simulink model "general_charger_2_precharge"  (R2013a)
settings: Solver=ode23  StartTime=0  StopTime=1.5  RelTol=1e-3
PreLoadFcn:
  | Ts =5e-6;
values from neighbouring files (symbols this model uses):
  ac_volt = 169    [charger_init.m]    (also in charger_init_simpl.m)
  acdc_on_time = 0.2    [charger_init.m]    (also in charger_init_simpl.m = 0)
  Cdc = 2e-3    (= 0.002)    [charger_init.m]    (also in charger_init_simpl.m)
  dcAd = dcinvexp*(eye(dcnstates) + (Ts/2)*dcAc)    [charger_init.m]    (also in charger_init_simpl.m)
  dcBd = dcinvexp*dcBc    [charger_init.m]    (also in charger_init_simpl.m)
  dcCd = dcCc*dcinvexp*Ts    [charger_init.m]    (also in charger_init_simpl.m)
  dcDd = dcCc*dcinvexp*dcBc*(Ts/2) + dcDc    [charger_init.m]    (also in charger_init_simpl.m)
  ESRCd = 70e-3    (= 0.07)    [charger_init.m]    (also in charger_init_simpl.m)
  ESRLdcdc = 0.1    [charger_init.m]    (also in charger_init_simpl.m)
  ESRLin = 0.2    [charger_init.m]    (also in charger_init_simpl.m = 0.1)
  Ldcdc = 1.3e-3    (= 0.0013)    [charger_init.m]    (also in charger_init_simpl.m = 0.0014)
  Lin = 1.5e-3    (= 0.0015)    [charger_init.m]    (also in charger_init_simpl.m = 0.001)
  P = 1.92e3    (= 1920)    [charger_init.m]    (also in charger_init_simpl.m)
  pre_charge_off = 0.2    [charger_init.m]
  pre_charge_r = 10    [charger_init.m]    (also in charger_init_simpl.m = 6)
  pre_charge_ramp = (dc_volt - Vdcmin)/(acdc_ramp_end_time - acdc_on_time)    (= 336.666666667)    [charger_init.m]    (also in charger_init_simpl.m = (dc_volt - Vdcmin)/(acdc_ramp_end_time - acdc_on_time))
  Q = 0    [charger_init.m]    (also in charger_init_simpl.m)
  Rbatt = 0.20    (= 0.2)    [charger_init.m]    (also in charger_init_simpl.m = 0.1)
  switch_Ts = 5e-5    (= 5e-05)    [charger_init.m]    (also in charger_init_simpl.m)
  sys_Ts = 5e-6    (= 5e-06)    [charger_init.m]    (also in charger_init_simpl.m)
  Vdcmin = ac_volt + 10    (= 179)    [charger_init.m]    (also in charger_init_simpl.m)
  voc = 105    [charger_init.m]    (also in charger_init_simpl.m)
undefined symbols (not defined in the file or in its folder): cpi
undefined symbols (not defined in the file): active_power_on, Ad, Bd, Cd, dc_volt, dcdc_cc_ref, dcdc_cv_ref, dcdc_iki, dcdc_ikp, dcdc_on, dcdc_vki, dcdc_vkp, Dd, dq_id_ki, dq_id_kp, dq_iq_ki, dq_iq_kp, dq_vdc_ki, dq_vdc_kp, dqQ_ki, dqQ_kp, P_ki, P_kp, pi_iac_ki, pi_iac_kp, pi_vdc_ki, pi_vdc_kp, piQ_ki, piQ_kp, pr_iac_kp, pr_pr_ki, pr_pr_kp, pr_vdc_ki, pr_vdc_kp, reactive_power_on
libraries: simulink_extras x165, powerlib x64, simulink x35, powerlib_meascontrol x11
(part 4 of 7)

== system general_charger_2_precharge/Measurements/THD/discrete low pass filter1/Ad(2,2) ==
  in : Inport
  Constant1 : Constant  Value=variable
  Product1 : Product
  Scope1 : Scope  NumInputPorts=2
      settings: YMin=-5~-5  YMax=5~5
  q rounder16 : Subsystem  mask{q=nQ, range=maxRange}
      mask prompts: q "q value"; range "q range"
  out : Outport
  wires:
  q rounder16/1(out) -> Product1/1, Scope1/2
  Constant1/1 -> Scope1/1, q rounder16/1(in)
  Product1/1 -> out/1
  in/1 -> Product1/2

== system general_charger_2_precharge/Measurements/THD/discrete low pass filter1/Ad(2,3) ==
  in : Inport
  Constant1 : Constant  Value=variable
  Product1 : Product
  Scope1 : Scope  NumInputPorts=2
      settings: YMin=-5~-5  YMax=5~5
  q rounder16 : Subsystem  mask{q=nQ, range=maxRange}
      mask prompts: q "q value"; range "q range"
  out : Outport
  wires:
  q rounder16/1(out) -> Product1/1, Scope1/2
  Constant1/1 -> Scope1/1, q rounder16/1(in)
  Product1/1 -> out/1
  in/1 -> Product1/2

== system general_charger_2_precharge/Measurements/THD/discrete low pass filter1/Ad(3,1) ==
  in : Inport
  Constant1 : Constant  Value=variable
  Product1 : Product
  Scope1 : Scope  NumInputPorts=2
      settings: YMin=-5~-5  YMax=5~5
  q rounder16 : Subsystem  mask{q=nQ, range=maxRange}
      mask prompts: q "q value"; range "q range"
  out : Outport
  wires:
  q rounder16/1(out) -> Product1/1, Scope1/2
  Constant1/1 -> Scope1/1, q rounder16/1(in)
  Product1/1 -> out/1
  in/1 -> Product1/2

== system general_charger_2_precharge/Measurements/THD/discrete low pass filter1/Ad(3,2) ==
  in : Inport
  Constant1 : Constant  Value=variable
  Product1 : Product
  Scope1 : Scope  NumInputPorts=2
      settings: YMin=-5~-5  YMax=5~5
  q rounder16 : Subsystem  mask{q=nQ, range=maxRange}
      mask prompts: q "q value"; range "q range"
  out : Outport
  wires:
  q rounder16/1(out) -> Product1/1, Scope1/2
  Constant1/1 -> Scope1/1, q rounder16/1(in)
  Product1/1 -> out/1
  in/1 -> Product1/2

== system general_charger_2_precharge/Measurements/THD/discrete low pass filter1/Ad(3,3) ==
  in : Inport
  Constant1 : Constant  Value=variable
  Product1 : Product
  Scope1 : Scope  NumInputPorts=2
      settings: YMin=-5~-5  YMax=5~5
  q rounder16 : Subsystem  mask{q=nQ, range=maxRange}
      mask prompts: q "q value"; range "q range"
  out : Outport
  wires:
  q rounder16/1(out) -> Product1/1, Scope1/2
  Constant1/1 -> Scope1/1, q rounder16/1(in)
  Product1/1 -> out/1
  in/1 -> Product1/2

== system general_charger_2_precharge/Measurements/THD/discrete low pass filter1/Bd(1) ==
  in : Inport
  Constant1 : Constant  Value=variable
  Product1 : Product
  q rounder16 : Subsystem  mask{q=nQ, range=maxRange}
      mask prompts: q "q value"; range "q range"
  out : Outport
  wires:
  q rounder16/1(out) -> Product1/1
  Constant1/1 -> q rounder16/1(in)
  Product1/1 -> out/1
  in/1 -> Product1/2

== system general_charger_2_precharge/Measurements/THD/discrete low pass filter1/Bd(2) ==
  in : Inport
  Constant1 : Constant  Value=variable
  Product1 : Product
  q rounder16 : Subsystem  mask{q=nQ, range=maxRange}
      mask prompts: q "q value"; range "q range"
  out : Outport
  wires:
  q rounder16/1(out) -> Product1/1
  Constant1/1 -> q rounder16/1(in)
  Product1/1 -> out/1
  in/1 -> Product1/2

== system general_charger_2_precharge/Measurements/THD/discrete low pass filter1/Bd(3) ==
  in : Inport
  Constant1 : Constant  Value=variable
  Product1 : Product
  q rounder16 : Subsystem  mask{q=nQ, range=maxRange}
      mask prompts: q "q value"; range "q range"
  out : Outport
  wires:
  q rounder16/1(out) -> Product1/1
  Constant1/1 -> q rounder16/1(in)
  Product1/1 -> out/1
  in/1 -> Product1/2

== system general_charger_2_precharge/Measurements/THD/discrete low pass filter1/Cd(1) ==
  in : Inport
  Constant1 : Constant  Value=variable
  Product1 : Product
  q rounder16 : Subsystem  mask{q=nQ, range=maxRange}
      mask prompts: q "q value"; range "q range"
  out : Outport
  wires:
  q rounder16/1(out) -> Product1/1
  Constant1/1 -> q rounder16/1(in)
  Product1/1 -> out/1
  in/1 -> Product1/2

== system general_charger_2_precharge/Measurements/THD/discrete low pass filter1/Cd(2) ==
  in : Inport
  Constant1 : Constant  Value=variable
  Product1 : Product
  q rounder16 : Subsystem  mask{q=nQ, range=maxRange}
      mask prompts: q "q value"; range "q range"
  out : Outport
  wires:
  q rounder16/1(out) -> Product1/1
  Constant1/1 -> q rounder16/1(in)
  Product1/1 -> out/1
  in/1 -> Product1/2

== system general_charger_2_precharge/Measurements/THD/discrete low pass filter1/Cd(3) ==
  in : Inport
  Constant1 : Constant  Value=variable
  Product1 : Product
  q rounder16 : Subsystem  mask{q=nQ, range=maxRange}
      mask prompts: q "q value"; range "q range"
  out : Outport
  wires:
  q rounder16/1(out) -> Product1/1
  Constant1/1 -> q rounder16/1(in)
  Product1/1 -> out/1
  in/1 -> Product1/2

== system general_charger_2_precharge/Measurements/THD/discrete low pass filter1/Dd ==
  in : Inport
  Constant1 : Constant  Value=variable
  Product1 : Product
  Scope1 : Scope  NumInputPorts=2
      settings: YMin=-5~-5  YMax=5~5
  q rounder16 : Subsystem  mask{q=nQ, range=maxRange}
      mask prompts: q "q value"; range "q range"
  out : Outport
  wires:
  q rounder16/1(out) -> Product1/1, Scope1/2
  Constant1/1 -> Scope1/1, q rounder16/1(in)
  Product1/1 -> out/1
  in/1 -> Product1/2

== system general_charger_2_precharge/Measurements/THD/discrete low pass filter1/q rounder1 ==
  in : Inport
  Gain9 : Gain  Gain=2^-q
  Idealized ADC quantizer : simulink_extras/Additional Discrete/Idealized ADC quantizer  NumberOfConverterBits=32  Vmin=-range  Vmax=range  OutputDataType=double  OutputNegativeValues=on
  out : Outport
  wires:
  in/1 -> Idealized ADC quantizer/1
  Idealized ADC quantizer/1 -> Gain9/1
  Gain9/1 -> out/1

== system general_charger_2_precharge/Measurements/THD/discrete low pass filter1/q rounder10 ==
  in : Inport
  Gain9 : Gain  Gain=2^-q
  Idealized ADC quantizer : simulink_extras/Additional Discrete/Idealized ADC quantizer  NumberOfConverterBits=32  Vmin=-range  Vmax=range  OutputDataType=double  OutputNegativeValues=on
  out : Outport
  wires:
  in/1 -> Idealized ADC quantizer/1
  Idealized ADC quantizer/1 -> Gain9/1
  Gain9/1 -> out/1

== system general_charger_2_precharge/Measurements/THD/discrete low pass filter1/q rounder11 ==
  in : Inport
  Gain9 : Gain  Gain=2^-q
  Idealized ADC quantizer : simulink_extras/Additional Discrete/Idealized ADC quantizer  NumberOfConverterBits=32  Vmin=-range  Vmax=range  OutputDataType=double  OutputNegativeValues=on
  out : Outport
  wires:
  in/1 -> Idealized ADC quantizer/1
  Idealized ADC quantizer/1 -> Gain9/1
  Gain9/1 -> out/1

== system general_charger_2_precharge/Measurements/THD/discrete low pass filter1/q rounder12 ==
  in : Inport
  Gain9 : Gain  Gain=2^-q
  Idealized ADC quantizer : simulink_extras/Additional Discrete/Idealized ADC quantizer  NumberOfConverterBits=32  Vmin=-range  Vmax=range  OutputDataType=double  OutputNegativeValues=on
  out : Outport
  wires:
  in/1 -> Idealized ADC quantizer/1
  Idealized ADC quantizer/1 -> Gain9/1
  Gain9/1 -> out/1

== system general_charger_2_precharge/Measurements/THD/discrete low pass filter1/q rounder13 ==
  in : Inport
  Gain9 : Gain  Gain=2^-q
  Idealized ADC quantizer : simulink_extras/Additional Discrete/Idealized ADC quantizer  NumberOfConverterBits=32  Vmin=-range  Vmax=range  OutputDataType=double  OutputNegativeValues=on
  out : Outport
  wires:
  in/1 -> Idealized ADC quantizer/1
  Idealized ADC quantizer/1 -> Gain9/1
  Gain9/1 -> out/1

== system general_charger_2_precharge/Measurements/THD/discrete low pass filter1/q rounder14 ==
  in : Inport
  Gain9 : Gain  Gain=2^-q
  Idealized ADC quantizer : simulink_extras/Additional Discrete/Idealized ADC quantizer  NumberOfConverterBits=32  Vmin=-range  Vmax=range  OutputDataType=double  OutputNegativeValues=on
  out : Outport
  wires:
  in/1 -> Idealized ADC quantizer/1
  Idealized ADC quantizer/1 -> Gain9/1
  Gain9/1 -> out/1

== system general_charger_2_precharge/Measurements/THD/discrete low pass filter1/q rounder15 ==
  in : Inport
  Gain9 : Gain  Gain=2^-q
  Idealized ADC quantizer : simulink_extras/Additional Discrete/Idealized ADC quantizer  NumberOfConverterBits=32  Vmin=-range  Vmax=range  OutputDataType=double  OutputNegativeValues=on
  out : Outport
  wires:
  in/1 -> Idealized ADC quantizer/1
  Idealized ADC quantizer/1 -> Gain9/1
  Gain9/1 -> out/1

== system general_charger_2_precharge/Measurements/THD/discrete low pass filter1/q rounder16 ==
  in : Inport
  Gain9 : Gain  Gain=2^-q
  Idealized ADC quantizer : simulink_extras/Additional Discrete/Idealized ADC quantizer  NumberOfConverterBits=32  Vmin=-range  Vmax=range  OutputDataType=double  OutputNegativeValues=on
  out : Outport
  wires:
  in/1 -> Idealized ADC quantizer/1
  Idealized ADC quantizer/1 -> Gain9/1
  Gain9/1 -> out/1

== system general_charger_2_precharge/Measurements/THD/discrete low pass filter1/q rounder17 ==
  in : Inport
  Gain9 : Gain  Gain=2^-q
  Idealized ADC quantizer : simulink_extras/Additional Discrete/Idealized ADC quantizer  NumberOfConverterBits=32  Vmin=-range  Vmax=range  OutputDataType=double  OutputNegativeValues=on
  out : Outport
  wires:
  in/1 -> Idealized ADC quantizer/1
  Idealized ADC quantizer/1 -> Gain9/1
  Gain9/1 -> out/1

== system general_charger_2_precharge/Measurements/THD/discrete low pass filter1/q rounder2 ==
  in : Inport
  Gain9 : Gain  Gain=2^-q
  Idealized ADC quantizer : simulink_extras/Additional Discrete/Idealized ADC quantizer  NumberOfConverterBits=32  Vmin=-range  Vmax=range  OutputDataType=double  OutputNegativeValues=on
  out : Outport
  wires:
  in/1 -> Idealized ADC quantizer/1
  Idealized ADC quantizer/1 -> Gain9/1
  Gain9/1 -> out/1

== system general_charger_2_precharge/Measurements/THD/discrete low pass filter1/q rounder3 ==
  in : Inport
  Gain9 : Gain  Gain=2^-q
  Idealized ADC quantizer : simulink_extras/Additional Discrete/Idealized ADC quantizer  NumberOfConverterBits=32  Vmin=-range  Vmax=range  OutputDataType=double  OutputNegativeValues=on
  out : Outport
  wires:
  in/1 -> Idealized ADC quantizer/1
  Idealized ADC quantizer/1 -> Gain9/1
  Gain9/1 -> out/1

== system general_charger_2_precharge/Measurements/THD/discrete low pass filter1/q rounder4 ==
  in : Inport
  Gain9 : Gain  Gain=2^-q
  Idealized ADC quantizer : simulink_extras/Additional Discrete/Idealized ADC quantizer  NumberOfConverterBits=32  Vmin=-range  Vmax=range  OutputDataType=double  OutputNegativeValues=on
  out : Outport
  wires:
  in/1 -> Idealized ADC quantizer/1
  Idealized ADC quantizer/1 -> Gain9/1
  Gain9/1 -> out/1

== system general_charger_2_precharge/Measurements/THD/discrete low pass filter1/q rounder5 ==
  in : Inport
  Gain9 : Gain  Gain=2^-q
  Idealized ADC quantizer : simulink_extras/Additional Discrete/Idealized ADC quantizer  NumberOfConverterBits=32  Vmin=-range  Vmax=range  OutputDataType=double  OutputNegativeValues=on
  out : Outport
  wires:
  in/1 -> Idealized ADC quantizer/1
  Idealized ADC quantizer/1 -> Gain9/1
  Gain9/1 -> out/1

== system general_charger_2_precharge/Measurements/THD/discrete low pass filter1/q rounder6 ==
  in : Inport
  Gain9 : Gain  Gain=2^-q
  Idealized ADC quantizer : simulink_extras/Additional Discrete/Idealized ADC quantizer  NumberOfConverterBits=32  Vmin=-range  Vmax=range  OutputDataType=double  OutputNegativeValues=on
  out : Outport
  wires:
  in/1 -> Idealized ADC quantizer/1
  Idealized ADC quantizer/1 -> Gain9/1
  Gain9/1 -> out/1

== system general_charger_2_precharge/Measurements/THD/discrete low pass filter1/q rounder7 ==
  in : Inport
  Gain9 : Gain  Gain=2^-q
  Idealized ADC quantizer : simulink_extras/Additional Discrete/Idealized ADC quantizer  NumberOfConverterBits=32  Vmin=-range  Vmax=range  OutputDataType=double  OutputNegativeValues=on
  out : Outport
  wires:
  in/1 -> Idealized ADC quantizer/1
  Idealized ADC quantizer/1 -> Gain9/1
  Gain9/1 -> out/1

== system general_charger_2_precharge/Measurements/THD/discrete low pass filter1/q rounder8 ==
  in : Inport
  Gain9 : Gain  Gain=2^-q
  Idealized ADC quantizer : simulink_extras/Additional Discrete/Idealized ADC quantizer  NumberOfConverterBits=32  Vmin=-range  Vmax=range  OutputDataType=double  OutputNegativeValues=on
  out : Outport
  wires:
  in/1 -> Idealized ADC quantizer/1
  Idealized ADC quantizer/1 -> Gain9/1
  Gain9/1 -> out/1

== system general_charger_2_precharge/Measurements/THD/discrete low pass filter1/q rounder9 ==
  in : Inport
  Gain9 : Gain  Gain=2^-q
  Idealized ADC quantizer : simulink_extras/Additional Discrete/Idealized ADC quantizer  NumberOfConverterBits=32  Vmin=-range  Vmax=range  OutputDataType=double  OutputNegativeValues=on
  out : Outport
  wires:
  in/1 -> Idealized ADC quantizer/1
  Idealized ADC quantizer/1 -> Gain9/1
  Gain9/1 -> out/1

== system general_charger_2_precharge/Measurements/discrete low pass filter1/Ad(1,1)/q rounder16 ==
  in : Inport
  Gain9 : Gain  Gain=2^-q
  Idealized ADC quantizer : simulink_extras/Additional Discrete/Idealized ADC quantizer  NumberOfConverterBits=32  Vmin=-range  Vmax=range  OutputDataType=double  OutputNegativeValues=on
  out : Outport
  wires:
  in/1 -> Idealized ADC quantizer/1
  Idealized ADC quantizer/1 -> Gain9/1
  Gain9/1 -> out/1

== system general_charger_2_precharge/Measurements/discrete low pass filter1/Ad(1,2)/q rounder16 ==
  in : Inport
  Gain9 : Gain  Gain=2^-q
  Idealized ADC quantizer : simulink_extras/Additional Discrete/Idealized ADC quantizer  NumberOfConverterBits=32  Vmin=-range  Vmax=range  OutputDataType=double  OutputNegativeValues=on
  out : Outport
  wires:
  in/1 -> Idealized ADC quantizer/1
  Idealized ADC quantizer/1 -> Gain9/1
  Gain9/1 -> out/1

== system general_charger_2_precharge/Measurements/discrete low pass filter1/Ad(1,3)/q rounder16 ==
  in : Inport
  Gain9 : Gain  Gain=2^-q
  Idealized ADC quantizer : simulink_extras/Additional Discrete/Idealized ADC quantizer  NumberOfConverterBits=32  Vmin=-range  Vmax=range  OutputDataType=double  OutputNegativeValues=on
  out : Outport
  wires:
  in/1 -> Idealized ADC quantizer/1
  Idealized ADC quantizer/1 -> Gain9/1
  Gain9/1 -> out/1

== system general_charger_2_precharge/Measurements/discrete low pass filter1/Ad(2,1)/q rounder16 ==
  in : Inport
  Gain9 : Gain  Gain=2^-q
  Idealized ADC quantizer : simulink_extras/Additional Discrete/Idealized ADC quantizer  NumberOfConverterBits=32  Vmin=-range  Vmax=range  OutputDataType=double  OutputNegativeValues=on
  out : Outport
  wires:
  in/1 -> Idealized ADC quantizer/1
  Idealized ADC quantizer/1 -> Gain9/1
  Gain9/1 -> out/1

== system general_charger_2_precharge/Measurements/discrete low pass filter1/Ad(2,2)/q rounder16 ==
  in : Inport
  Gain9 : Gain  Gain=2^-q
  Idealized ADC quantizer : simulink_extras/Additional Discrete/Idealized ADC quantizer  NumberOfConverterBits=32  Vmin=-range  Vmax=range  OutputDataType=double  OutputNegativeValues=on
  out : Outport
  wires:
  in/1 -> Idealized ADC quantizer/1
  Idealized ADC quantizer/1 -> Gain9/1
  Gain9/1 -> out/1

== system general_charger_2_precharge/Measurements/discrete low pass filter1/Ad(2,3)/q rounder16 ==
  in : Inport
  Gain9 : Gain  Gain=2^-q
  Idealized ADC quantizer : simulink_extras/Additional Discrete/Idealized ADC quantizer  NumberOfConverterBits=32  Vmin=-range  Vmax=range  OutputDataType=double  OutputNegativeValues=on
  out : Outport
  wires:
  in/1 -> Idealized ADC quantizer/1
  Idealized ADC quantizer/1 -> Gain9/1
  Gain9/1 -> out/1

== system general_charger_2_precharge/Measurements/discrete low pass filter1/Ad(3,1)/q rounder16 ==
  in : Inport
  Gain9 : Gain  Gain=2^-q
  Idealized ADC quantizer : simulink_extras/Additional Discrete/Idealized ADC quantizer  NumberOfConverterBits=32  Vmin=-range  Vmax=range  OutputDataType=double  OutputNegativeValues=on
  out : Outport
  wires:
  in/1 -> Idealized ADC quantizer/1
  Idealized ADC quantizer/1 -> Gain9/1
  Gain9/1 -> out/1

== system general_charger_2_precharge/Measurements/discrete low pass filter1/Ad(3,2)/q rounder16 ==
  in : Inport
  Gain9 : Gain  Gain=2^-q
  Idealized ADC quantizer : simulink_extras/Additional Discrete/Idealized ADC quantizer  NumberOfConverterBits=32  Vmin=-range  Vmax=range  OutputDataType=double  OutputNegativeValues=on
  out : Outport
  wires:
  in/1 -> Idealized ADC quantizer/1
  Idealized ADC quantizer/1 -> Gain9/1
  Gain9/1 -> out/1

== system general_charger_2_precharge/Measurements/discrete low pass filter1/Ad(3,3)/q rounder16 ==
  in : Inport
  Gain9 : Gain  Gain=2^-q
  Idealized ADC quantizer : simulink_extras/Additional Discrete/Idealized ADC quantizer  NumberOfConverterBits=32  Vmin=-range  Vmax=range  OutputDataType=double  OutputNegativeValues=on
  out : Outport
  wires:
  in/1 -> Idealized ADC quantizer/1
  Idealized ADC quantizer/1 -> Gain9/1
  Gain9/1 -> out/1

== system general_charger_2_precharge/Measurements/discrete low pass filter1/Bd(1)/q rounder16 ==
  in : Inport
  Gain9 : Gain  Gain=2^-q
  Idealized ADC quantizer : simulink_extras/Additional Discrete/Idealized ADC quantizer  NumberOfConverterBits=32  Vmin=-range  Vmax=range  OutputDataType=double  OutputNegativeValues=on
  out : Outport
  wires:
  in/1 -> Idealized ADC quantizer/1
  Idealized ADC quantizer/1 -> Gain9/1
  Gain9/1 -> out/1

== system general_charger_2_precharge/Measurements/discrete low pass filter1/Bd(2)/q rounder16 ==
  in : Inport
  Gain9 : Gain  Gain=2^-q
  Idealized ADC quantizer : simulink_extras/Additional Discrete/Idealized ADC quantizer  NumberOfConverterBits=32  Vmin=-range  Vmax=range  OutputDataType=double  OutputNegativeValues=on
  out : Outport
  wires:
  in/1 -> Idealized ADC quantizer/1
  Idealized ADC quantizer/1 -> Gain9/1
  Gain9/1 -> out/1

== system general_charger_2_precharge/Measurements/discrete low pass filter1/Bd(3)/q rounder16 ==
  in : Inport
  Gain9 : Gain  Gain=2^-q
  Idealized ADC quantizer : simulink_extras/Additional Discrete/Idealized ADC quantizer  NumberOfConverterBits=32  Vmin=-range  Vmax=range  OutputDataType=double  OutputNegativeValues=on
  out : Outport
  wires:
  in/1 -> Idealized ADC quantizer/1
  Idealized ADC quantizer/1 -> Gain9/1
  Gain9/1 -> out/1

== system general_charger_2_precharge/Measurements/discrete low pass filter1/Cd(1)/q rounder16 ==
  in : Inport
  Gain9 : Gain  Gain=2^-q
  Idealized ADC quantizer : simulink_extras/Additional Discrete/Idealized ADC quantizer  NumberOfConverterBits=32  Vmin=-range  Vmax=range  OutputDataType=double  OutputNegativeValues=on
  out : Outport
  wires:
  in/1 -> Idealized ADC quantizer/1
  Idealized ADC quantizer/1 -> Gain9/1
  Gain9/1 -> out/1

== system general_charger_2_precharge/Measurements/discrete low pass filter1/Cd(2)/q rounder16 ==
  in : Inport
  Gain9 : Gain  Gain=2^-q
  Idealized ADC quantizer : simulink_extras/Additional Discrete/Idealized ADC quantizer  NumberOfConverterBits=32  Vmin=-range  Vmax=range  OutputDataType=double  OutputNegativeValues=on
  out : Outport
  wires:
  in/1 -> Idealized ADC quantizer/1
  Idealized ADC quantizer/1 -> Gain9/1
  Gain9/1 -> out/1

== system general_charger_2_precharge/Measurements/discrete low pass filter1/Cd(3)/q rounder16 ==
  in : Inport
  Gain9 : Gain  Gain=2^-q
  Idealized ADC quantizer : simulink_extras/Additional Discrete/Idealized ADC quantizer  NumberOfConverterBits=32  Vmin=-range  Vmax=range  OutputDataType=double  OutputNegativeValues=on
  out : Outport
  wires:
  in/1 -> Idealized ADC quantizer/1
  Idealized ADC quantizer/1 -> Gain9/1
  Gain9/1 -> out/1

== system general_charger_2_precharge/Measurements/discrete low pass filter1/Dd/q rounder16 ==
  in : Inport
  Gain9 : Gain  Gain=2^-q
  Idealized ADC quantizer : simulink_extras/Additional Discrete/Idealized ADC quantizer  NumberOfConverterBits=32  Vmin=-range  Vmax=range  OutputDataType=double  OutputNegativeValues=on
  out : Outport
  wires:
  in/1 -> Idealized ADC quantizer/1
  Idealized ADC quantizer/1 -> Gain9/1
  Gain9/1 -> out/1

== system general_charger_2_precharge/control_stage/AC//DC Control/DQ Controller/AB-DQ Transform ==
  Va : Inport
  Ia : Inport  Port=2
  phi : Inport  Port=3
  AB->DQ : Subsystem  mask{abdq_f=60, abdq_Ts=switch_Ts}
      mask prompts: abdq_f "frequency"; abdq_Ts "Sample Time"
      mask init:
      | SpC=1/abdq_f/4/abdq_Ts;
      | RSpC=ceil(SpC);
  PLL : Subsystem  mask{pll_f=60, pll_Ts=switch_Ts, pll_ki=50, pll_kp=5}
      mask prompts: pll_f "frequency"; pll_Ts "Sample Time"; pll_ki "PI Integral Gain"; pll_kp "PI Proportional Gain"
  Vd : Outport
  Vq : Outport  Port=2
  Id : Outport  Port=3
  Iq : Outport  Port=4
  theta : Outport  Port=5
  wires:
  phi/1 -> AB->DQ/3(phi)
  Va/1 -> PLL/1(signal_in)
  Ia/1 -> AB->DQ/1(A)
  PLL/2(D) -> Vd/1
  PLL/3(Q) -> Vq/1
  PLL/1(angle_out) -> theta/1, AB->DQ/2(wt)
  AB->DQ/1(D) -> Id/1
  AB->DQ/2(Q) -> Iq/1

== system general_charger_2_precharge/control_stage/AC//DC Control/DQ Controller/DQ Controller Submodule ==
  note: id_error
  Vdc : Inport
  Vd : Inport  Port=2
  Id : Inport  Port=3
  Iq : Inport  Port=4
  Vwt : Inport  Port=5
  Add{1..2,6..7} (4 alike) : Sum  Inputs=-+
  Add3 : Sum  Inputs=+-
  Add4 : Sum  Inputs=+++
  Add5 : Sum  Inputs=+-
  Constant : Constant  Value=50
  Constant4 : Constant  Value=vdc
  DQ-->A : Subsystem
  Divide : Product  Inputs=*/
  Divide1 : Product  Inputs=/*
  Gain : Gain  Gain=2*pi*f*L
  Gain1 : Gain  Gain=R
  Gain2 : Gain  Gain=2*pi*f*L
  Gain3 : Gain  Gain=R
  PI1 : Subsystem  mask{ki=id_ki, kp=id_kp, Ts_pi=Ts, int_sat_up=500, int_sat_low=-500, pi_sat_up=500, pi_sat_low=-500}
      mask prompts: ki "Integral Gain"; kp "Proportional Gain"; Ts_pi "Sample Time"; int_sat_up "Integral Saturation Upper"; int_sat_low "Integral Saturation Lower"; pi_sat_up "PI Controller Saturation Upper"; pi_sat_low "PI Controller Saturation Lower"
      mask Display: disp('PI')
  PI2 : Subsystem  mask{ki=vdc_ki, kp=vdc_kp, Ts_pi=Ts, int_sat_up=500, int_sat_low=-500, pi_sat_up=500, pi_sat_low=-500}
      mask prompts: ki "Integral Gain"; kp "Proportional Gain"; Ts_pi "Sample Time"; int_sat_up "Integral Saturation Upper"; int_sat_low "Integral Saturation Lower"; pi_sat_up "PI Controller Saturation Upper"; pi_sat_low "PI Controller Saturation Lower"
      mask Display: disp('PI')
  PI3 : Subsystem  mask{ki=iq_ki, kp=iq_kp, Ts_pi=Ts, int_sat_up=500, int_sat_low=-500, pi_sat_up=500, pi_sat_low=-500}
      mask prompts: ki "Integral Gain"; kp "Proportional Gain"; Ts_pi "Sample Time"; int_sat_up "Integral Saturation Upper"; int_sat_low "Integral Saturation Lower"; pi_sat_up "PI Controller Saturation Upper"; pi_sat_low "PI Controller Saturation Lower"
      mask Display: disp('PI')
  Ramp : simulink/Sources/Ramp  slope=pre_charge_ramp  start=acdc_on_time  X0=Vdcmin
  Reactive Power Control Module : Subsystem
  Scope : Scope
      settings: SaveName=ScopeData12
  Switch : Switch  Threshold=50
  Switch1 : Switch  Threshold=vdc
  Va : Outport
  tag scope: nVd=global
  wires:
  Add2/1 -> PI2/1(in)  "dq_vdc_error"
  Add3/1 -> Gain1/1, Gain2/1, PI1/1(in)
  PI3/1(out) -> Add6/2  "iq_pi"
  Add4/1 -> Add5/1
  Gain/1 -> Add4/3
  Gain1/1 -> Add5/2
  PI2/1(out) -> Add3/1  "dq_vdc_pi"
  Add6/1 -> Add7/2
  Gain3/1 -> Add7/1
  Gain2/1 -> Add6/1
  DQ-->A/1(A) -> Va/1
  Constant/1 -> Switch/3
  Switch/1 -> Divide1/1, Divide/2
  Vd/1 -> [nVd], Add4/1
  Id/1 -> Add3/2
  Vwt/1 -> DQ-->A/3(wt)
  Add1/1 -> PI3/1(in), Gain3/1, Gain/1  "iq_error"
  Add7/1 -> Divide1/2  "iq_corr"
  Divide1/1 -> DQ-->A/2(Q)  "iq_corr_scale"
  Add5/1 -> Divide/1  "id_corr"
  Divide/1 -> DQ-->A/1(D)  "id_corr_scale"
  Iq/1 -> Add1/1
  Ramp/1 -> Switch1/3, Switch1/2
  Vdc/1 -> [dq_vdc], Add2/1
  Reactive Power Control Module/1(Iq_ref) -> Add1/2
  PI1/1(out) -> Add4/2
  [dq_vdc] -> Switch/1, Switch/2
  Constant4/1 -> Switch1/1  "vdc_ref"
  Switch1/1 -> Scope/1, Add2/2

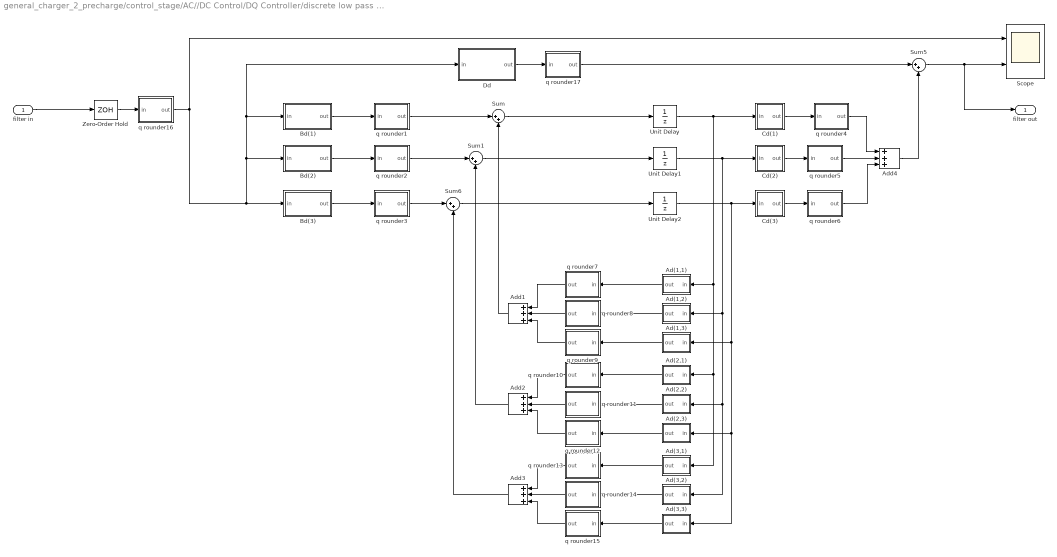
== system general_charger_2_precharge/control_stage/AC//DC Control/DQ Controller/discrete low pass filter1 ==
  filter in : Inport
  Ad(1,1) : Subsystem  mask{variable=Ad(1,1), nQ=29, maxRange=4}
      mask prompts: variable "state-space variable"; nQ "q value"; maxRange "max range"
      mask Display: disp(nQ)
  Ad(1,2) : Subsystem  mask{variable=Ad(1,2), nQ=23, maxRange=256}
      mask prompts: variable "state-space variable"; nQ "q value"; maxRange "max range"
      mask Display: disp(nQ)
  Ad(1,3) : Subsystem  mask{variable=Ad(1,3), nQ=14, maxRange=131072}
      mask prompts: variable "state-space variable"; nQ "q value"; maxRange "max range"
      mask Display: disp(nQ)
  Ad(2,1) : Subsystem  mask{variable=Ad(2,1), nQ=30, maxRange=2}
      mask prompts: variable "state-space variable"; nQ "q value"; maxRange "max range"
      mask Display: disp(nQ)
  Ad(2,2) : Subsystem  mask{variable=Ad(2,2), nQ=29, maxRange=4}
      mask prompts: variable "state-space variable"; nQ "q value"; maxRange "max range"
      mask Display: disp(nQ)
  Ad(2,3) : Subsystem  mask{variable=Ad(2,3), nQ=29, maxRange=4}
      mask prompts: variable "state-space variable"; nQ "q value"; maxRange "max range"
      mask Display: disp(nQ)
  Ad(3,1) : Subsystem  mask{variable=Ad(3,1), nQ=30, maxRange=2}
      mask prompts: variable "state-space variable"; nQ "q value"; maxRange "max range"
      mask Display: disp(nQ)
  Ad(3,2) : Subsystem  mask{variable=Ad(3,2), nQ=30, maxRange=2}
      mask prompts: variable "state-space variable"; nQ "q value"; maxRange "max range"
      mask Display: disp(nQ)
  Ad(3,3) : Subsystem  mask{variable=Ad(3,3), nQ=29, maxRange=4}
      mask prompts: variable "state-space variable"; nQ "q value"; maxRange "max range"
      mask Display: disp(nQ)
  Add{1..4} (4 alike) : Sum  Inputs=+++
  Bd(1) : Subsystem  mask{variable=Bd(1), nQ=29, maxRange=4}
      mask prompts: variable "state-space variable"; nQ "q value"; maxRange "max range"
      mask Display: disp(nQ)
  Bd(2) : Subsystem  mask{variable=Bd(2), nQ=30, maxRange=2}
      mask prompts: variable "state-space variable"; nQ "q value"; maxRange "max range"
      mask Display: disp(nQ)
  Bd(3) : Subsystem  mask{variable=Bd(3), nQ=30, maxRange=2}
      mask prompts: variable "state-space variable"; nQ "q value"; maxRange "max range"
      mask Display: disp(nQ)
  Cd(1) : Subsystem  mask{variable=Cd(1), nQ=30, maxRange=2}
      mask prompts: variable "state-space variable"; nQ "q value"; maxRange "max range"
      mask Display: disp(nQ)
  Cd(2) : Subsystem  mask{variable=Cd(2), nQ=23, maxRange=256}
      mask prompts: variable "state-space variable"; nQ "q value"; maxRange "max range"
      mask Display: disp(nQ)
  Cd(3) : Subsystem  mask{variable=Cd(3), nQ=15, maxRange=65536}
      mask prompts: variable "state-space variable"; nQ "q value"; maxRange "max range"
      mask Display: disp(nQ)
  Dd : Subsystem  mask{variable=Dd, nQ=30, maxRange=2}
      mask prompts: variable "state-space variable"; nQ "q value"; maxRange "max range"
      mask Display: disp(nQ)
  Scope : Scope  NumInputPorts=2
      settings: YMin=-5~-5  YMax=5~5  SaveName=ScopeData11
  Sum{,1,5..6} (4 alike) : Sum  Inputs=|++
  Unit Delay : UnitDelay  SampleTime=5e-5
  Unit Delay1 : UnitDelay  SampleTime=5e-5
  Unit Delay2 : UnitDelay  SampleTime=5e-5
  Zero-Order Hold : ZeroOrderHold  SampleTime=5e-5
  q rounder1 : Subsystem  mask{q=22, range=512}
      mask prompts: q "q value"; range "q range"
      mask Display: disp(q)
  q rounder10 : Subsystem  mask{q=30, range=2}
      mask prompts: q "q value"; range "q range"
      mask Display: disp(q)
  q rounder11 : Subsystem  mask{q=30, range=2}
      mask prompts: q "q value"; range "q range"
      mask Display: disp(q)
  q rounder12 : Subsystem  mask{q=30, range=2}
      mask prompts: q "q value"; range "q range"
      mask Display: disp(q)
  q rounder13 : Subsystem  mask{q=30, range=2}
      mask prompts: q "q value"; range "q range"
      mask Display: disp(q)
  q rounder14 : Subsystem  mask{q=30, range=2}
      mask prompts: q "q value"; range "q range"
      mask Display: disp(q)
  q rounder15 : Subsystem  mask{q=30, range=2}
      mask prompts: q "q value"; range "q range"
      mask Display: disp(q)
  q rounder16 : Subsystem  mask{q=19, range=4096}
      mask prompts: q "q value"; range "q range"
      mask Display: disp(q)
  q rounder17 : Subsystem  mask{q=30, range=2}
      mask prompts: q "q value"; range "q range"
      mask Display: disp(q)
  q rounder2 : Subsystem  mask{q=30, range=2}
      mask prompts: q "q value"; range "q range"
      mask Display: disp(q)
  q rounder3 : Subsystem  mask{q=30, range=2}
      mask prompts: q "q value"; range "q range"
      mask Display: disp(q)
  q rounder4 : Subsystem  mask{q=19, range=4096}
      mask prompts: q "q value"; range "q range"
      mask Display: disp(q)
  q rounder5 : Subsystem  mask{q=19, range=4096}
      mask prompts: q "q value"; range "q range"
      mask Display: disp(q)
  q rounder6 : Subsystem  mask{q=19, range=4096}
      mask prompts: q "q value"; range "q range"
      mask Display: disp(q)
  q rounder7 : Subsystem  mask{q=22, range=512}
      mask prompts: q "q value"; range "q range"
      mask Display: disp(q)
  q rounder8 : Subsystem  mask{q=22, range=512}
      mask prompts: q "q value"; range "q range"
      mask Display: disp(q)
  q rounder9 : Subsystem  mask{q=22, range=512}
      mask prompts: q "q value"; range "q range"
      mask Display: disp(q)
  filter out : Outport
  wires:
  Sum/1 -> Unit Delay/1
  Sum1/1 -> Unit Delay1/1
  Unit Delay/1 -> Ad(3,1)/1(in), Ad(2,1)/1(in), Ad(1,1)/1(in), Cd(1)/1(in)
  Unit Delay1/1 -> Ad(3,2)/1(in), Ad(2,2)/1(in), Ad(1,2)/1(in), Cd(2)/1(in)
  Dd/1(out) -> q rounder17/1(in)
  Sum5/1 -> filter out/1, Scope/2
  Zero-Order Hold/1 -> q rounder16/1(in)
  Sum6/1 -> Unit Delay2/1
  Unit Delay2/1 -> Ad(1,3)/1(in), Ad(3,3)/1(in), Ad(2,3)/1(in), Cd(3)/1(in)
  Ad(1,2)/1(out) -> q rounder8/1(in)
  Ad(1,1)/1(out) -> q rounder7/1(in)
  Ad(2,1)/1(out) -> q rounder10/1(in)
  Ad(2,3)/1(out) -> q rounder12/1(in)
  Ad(2,2)/1(out) -> q rounder11/1(in)
  Ad(3,2)/1(out) -> q rounder14/1(in)
  Ad(3,1)/1(out) -> q rounder13/1(in)
  Ad(3,3)/1(out) -> q rounder15/1(in)
  Add2/1 -> Sum1/2
  Add3/1 -> Sum6/2
  q rounder2/1(out) -> Sum1/1
  q rounder3/1(out) -> Sum6/1
  q rounder4/1(out) -> Add4/1
  q rounder5/1(out) -> Add4/2
  q rounder6/1(out) -> Add4/3
  q rounder7/1(out) -> Add1/1
  q rounder8/1(out) -> Add1/2
  q rounder9/1(out) -> Add1/3
  q rounder10/1(out) -> Add2/1
  q rounder11/1(out) -> Add2/2
  q rounder12/1(out) -> Add2/3
  q rounder13/1(out) -> Add3/1
  q rounder14/1(out) -> Add3/2
  q rounder15/1(out) -> Add3/3
  Bd(1)/1(out) -> q rounder1/1(in)
  Cd(1)/1(out) -> q rounder4/1(in)
  Bd(2)/1(out) -> q rounder2/1(in)
  Bd(3)/1(out) -> q rounder3/1(in)
  Cd(3)/1(out) -> q rounder6/1(in)
  Cd(2)/1(out) -> q rounder5/1(in)
  Ad(1,3)/1(out) -> q rounder9/1(in)
  q rounder16/1(out) -> Scope/1, Bd(3)/1(in), Bd(2)/1(in), Dd/1(in), Bd(1)/1(in)
  q rounder17/1(out) -> Sum5/1
  Add4/1 -> Sum5/2
  Add1/1 -> Sum/2
  q rounder1/1(out) -> Sum/1
  filter in/1 -> Zero-Order Hold/1

== system general_charger_2_precharge/control_stage/AC//DC Control/PI Controller/PI Reactive Power Controller ==
  vac in : Inport
  Add2 : Sum
  Add8 : Sum  Inputs=+-
  Constant2 : Constant  Value=Q
  Constant3 : Constant  Value=0
  Constant4 : Constant  Value=334
  PI2 : Subsystem  mask{ki=piQ_ki, kp=piQ_kp, Ts_pi=Ts, int_sat_up=inf, int_sat_low=-inf, pi_sat_up=inf, pi_sat_low=-inf, pi_on=turn_on}
      mask prompts: ki "Integral Gain"; kp "Proportional Gain"; Ts_pi "Sample Time"; int_sat_up "Integral Saturation Upper"; int_sat_low "Integral Saturation Lower"; pi_sat_up "PI Controller Saturation Upper"; pi_sat_low "PI Controller Saturation Lower"; pi_on "PI Controller Turn on Time, s"
      mask Display: disp('PI')
  Step1 : Step  Time=turn_on  SampleTime=0
  Switch3 : Switch  Threshold=0.5
  Variable Integer Delay : Delay  DelayLengthSource=Input port  DelayLengthUpperLimit=600  InitialCondition=334  SampleTime=switch_Ts
      settings: InputPortMap=u0,p1
  vac shifted : Outport
  wires:
  Add2/1 -> Variable Integer Delay/2
  Step1/1 -> Switch3/2
  [Qpower] -> Add8/2
  Constant2/1 -> Add8/1
  Variable Integer Delay/1 -> vac shifted/1
  Constant4/1 -> Add2/1
  PI2/1(out) -> Add2/2
  Constant3/1 -> Switch3/3
  Switch3/1 -> PI2/1(in)
  Add8/1 -> Switch3/1
  vac in/1 -> Variable Integer Delay/1

== system general_charger_2_precharge/control_stage/AC//DC Control/PI Controller/PI3 ==
  in : Inport
  Add1 : Sum
  Add2 : Sum
  Ki : Gain  Gain=ki
  Kp : Gain  Gain=kp
  Tappe : simulink/Discrete/Tapped Delay  vinit=0.0  samptime=Ts_pi  NumDelays=1  DelayOrder=Oldest  includeCurrent=off
  Ts : Gain  Gain=Ts_pi
  integral saturation : Saturate  UpperLimit=int_sat_up  LowerLimit=int_sat_low  SampleTime=Ts_pi
  pi controller saturation : Saturate  UpperLimit=pi_sat_up  LowerLimit=pi_sat_low  SampleTime=Ts_pi
  out : Outport
  wires:
  Ts/1 -> Ki/1
  in/1 -> Kp/1, Ts/1  "vdc_error"
  Add1/1 -> integral saturation/1  "vdc_int_pi"
  Kp/1 -> Add2/2  "vdc_kp_pi"
  pi controller saturation/1 -> out/1
  Tappe/1 -> Add1/1
  Add2/1 -> pi controller saturation/1  "vdc_pi"
  Ki/1 -> Add1/2
  integral saturation/1 -> Add2/1, Tappe/1

== system general_charger_2_precharge/control_stage/AC//DC Control/PI Controller/PI4 ==
  in : Inport
  Add1 : Sum
  Add2 : Sum
  Ki : Gain  Gain=ki
  Kp : Gain  Gain=kp
  Tappe : simulink/Discrete/Tapped Delay  vinit=0.0  samptime=Ts_pi  NumDelays=1  DelayOrder=Oldest  includeCurrent=off
  Ts : Gain  Gain=Ts_pi
  integral saturation : Saturate  UpperLimit=int_sat_up  LowerLimit=int_sat_low  SampleTime=Ts_pi
  pi controller saturation : Saturate  UpperLimit=pi_sat_up  LowerLimit=pi_sat_low  SampleTime=Ts_pi
  out : Outport
  wires:
  Ts/1 -> Ki/1
  in/1 -> Kp/1, Ts/1  "vdc_error"
  Add1/1 -> integral saturation/1  "vdc_int_pi"
  Kp/1 -> Add2/2  "vdc_kp_pi"
  pi controller saturation/1 -> out/1
  Tappe/1 -> Add1/1
  Add2/1 -> pi controller saturation/1  "vdc_pi"
  Ki/1 -> Add1/2
  integral saturation/1 -> Add2/1, Tappe/1

== system general_charger_2_precharge/control_stage/AC//DC Control/PR Controller/PI Reactive Power Controller ==
  vac in : Inport
  Add2 : Sum
  Add8 : Sum  Inputs=+-
  Constant2 : Constant  Value=Q
  Constant3 : Constant  Value=0
  Constant4 : Constant  Value=334
  PI2 : Subsystem  mask{ki=piQ_ki, kp=piQ_kp, Ts_pi=Ts, int_sat_up=inf, int_sat_low=-inf, pi_sat_up=inf, pi_sat_low=-inf, pi_on=turn_on}
      mask prompts: ki "Integral Gain"; kp "Proportional Gain"; Ts_pi "Sample Time"; int_sat_up "Integral Saturation Upper"; int_sat_low "Integral Saturation Lower"; pi_sat_up "PI Controller Saturation Upper"; pi_sat_low "PI Controller Saturation Lower"; pi_on "PI Controller Turn on Time, s"
      mask Display: disp('PI')
  Scope : Scope  NumInputPorts=4
      settings: YMin=334~-1~-1~-28500  YMax=334~1~1~-25000  SaveName=ScopeData7
  Step1 : Step  Time=turn_on  SampleTime=0
  Switch3 : Switch  Threshold=0.5
  Variable Integer Delay : Delay  DelayLengthSource=Input port  DelayLengthUpperLimit=600  InitialCondition=334  SampleTime=switch_Ts
      settings: InputPortMap=u0,p1
  vac shifted : Outport
  wires:
  Add2/1 -> Scope/1, Variable Integer Delay/2
  Step1/1 -> Switch3/2
  [Qpower] -> Add8/2
  Constant2/1 -> Add8/1
  Variable Integer Delay/1 -> vac shifted/1
  Constant4/1 -> Add2/1
  PI2/1(out) -> Scope/2, Add2/2
  Constant3/1 -> Switch3/3
  Switch3/1 -> Scope/3, PI2/1(in)
  Add8/1 -> Scope/4, Switch3/1
  vac in/1 -> Variable Integer Delay/1

== system general_charger_2_precharge/control_stage/AC//DC Control/PR Controller/PI2 ==
  in : Inport
  Add1 : Sum
  Add2 : Sum
  Ki : Gain  Gain=ki
  Kp : Gain  Gain=kp
  Tappe : simulink/Discrete/Tapped Delay  vinit=0.0  samptime=Ts_pi  NumDelays=1  DelayOrder=Oldest  includeCurrent=off
  Ts : Gain  Gain=Ts_pi
  integral saturation : Saturate  UpperLimit=int_sat_up  LowerLimit=int_sat_low  SampleTime=Ts_pi
  pi controller saturation : Saturate  UpperLimit=pi_sat_up  LowerLimit=pi_sat_low  SampleTime=Ts_pi
  out : Outport
  wires:
  Ts/1 -> Ki/1
  in/1 -> Kp/1, Ts/1  "vdc_error"
  Add1/1 -> integral saturation/1  "vdc_int_pi"
  Kp/1 -> Add2/2  "vdc_kp_pi"
  pi controller saturation/1 -> out/1
  Tappe/1 -> Add1/1
  Add2/1 -> pi controller saturation/1  "vdc_pi"
  Ki/1 -> Add1/2
  integral saturation/1 -> Add2/1, Tappe/1

== system general_charger_2_precharge/control_stage/AC//DC Control/PR Controller/PR Controller ==
  vac : Inport
  iac error : Inport  Port=2
  Add1 : Sum
  Add4 : Sum
  Gain : Gain  Gain=2
  Gain1 : Gain  Gain=iac_kp
  PI3 : Subsystem  mask{ki=pr_ki, kp=pr_kp, Ts_pi=Ts, int_sat_up=500, int_sat_low=-500, pi_sat_up=500, pi_sat_low=-500}
      mask prompts: ki "Integral Gain"; kp "Proportional Gain"; Ts_pi "Sample Time"; int_sat_up "Integral Saturation Upper"; int_sat_low "Integral Saturation Lower"; pi_sat_up "PI Controller Saturation Upper"; pi_sat_low "PI Controller Saturation Lower"
      mask Display: disp('PI')
  PI4 : Subsystem  mask{ki=pr_ki, kp=pr_kp, Ts_pi=Ts, int_sat_up=500, int_sat_low=-500, pi_sat_up=500, pi_sat_low=-500}
      mask prompts: ki "Integral Gain"; kp "Proportional Gain"; Ts_pi "Sample Time"; int_sat_up "Integral Saturation Upper"; int_sat_low "Integral Saturation Lower"; pi_sat_up "PI Controller Saturation Upper"; pi_sat_low "PI Controller Saturation Lower"
      mask Display: disp('PI')
  PLL : Subsystem  mask{pll_f=60, pll_Ts=switch_Ts, pll_ki=50, pll_kp=5}
      mask prompts: pll_f "frequency"; pll_Ts "Sample Time"; pll_ki "PI Integral Gain"; pll_kp "PI Proportional Gain"
  Product{,3..5} (4 alike) : Product
  Scope : Scope  NumInputPorts=4
      settings: YMin=-5~-5~-5~-5  YMax=5~5~5~5
  Terminator : Terminator
  Terminator1 : Terminator
  Trigonometric Function : Trigonometry  SampleTime=switch_Ts
  Trigonometric Function1 : Trigonometry  Operator=cos  SampleTime=switch_Ts
  output : Outport
  wires:
  Product3/1 -> PI4/1(in)
  Product/1 -> PI3/1(in)
  PI3/1(out) -> Product5/1
  Product5/1 -> Add4/2
  PLL/3(Q) -> Terminator1/1
  PLL/2(D) -> Terminator/1
  PLL/1(angle_out) -> Product4/1, Trigonometric Function/1, Trigonometric Function1/1
  Add4/1 -> Gain/1
  Trigonometric Function/1 -> Product3/1
  Product4/1 -> Scope/1, Add4/1
  Trigonometric Function1/1 -> Product5/2, Product/1
  iac error/1 -> Gain1/1, Product/2, Product3/2
  PI4/1(out) -> Product4/2
  vac/1 -> PLL/1(signal_in)
  Gain1/1 -> Scope/3, Add1/2
  Add1/1 -> Scope/4, output/1
  Gain/1 -> Scope/2, Add1/1

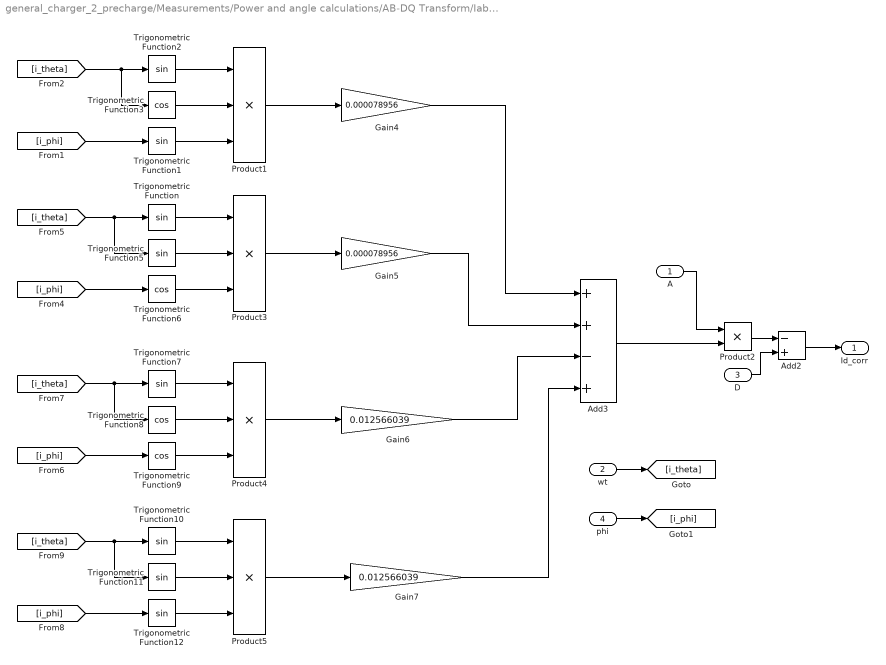
== system general_charger_2_precharge/Measurements/Power and angle calculations/AB-DQ Transform/Iab_dq/Id Discretization Error Correction ==
  A : Inport
  wt : Inport  Port=2
  D : Inport  Port=3
  phi : Inport  Port=4
  Add2 : Sum  Inputs=-+
  Add3 : Sum  Inputs=++-+
  Gain4 : Gain  Gain=0.000078956
  Gain5 : Gain  Gain=0.000078956
  Gain6 : Gain  Gain=0.012566039
  Gain7 : Gain  Gain=0.012566039
  Product{1,3..5} (4 alike) : Product  Inputs=3
  Product2 : Product
  Trigonometric Function{,1..2,5,7,10..12} (8 alike) : Trigonometry
  Trigonometric Function{3,6,8..9} (4 alike) : Trigonometry  Operator=cos
  Id_corr : Outport
  wires:
  Add2/1 -> Id_corr/1
  Product2/1 -> Add2/1
  D/1 -> Add2/2
  A/1 -> Product2/1
  wt/1 -> [i_theta]
  phi/1 -> [i_phi]
  [i_theta] -> Trigonometric Function3/1, Trigonometric Function2/1
  [i_phi] -> Trigonometric Function1/1
  Trigonometric Function1/1 -> Product1/3
  Trigonometric Function2/1 -> Product1/1
  Trigonometric Function3/1 -> Product1/2
  Product1/1 -> Gain4/1
  [i_theta] -> Trigonometric Function5/1, Trigonometric Function/1
  [i_phi] -> Trigonometric Function6/1
  Trigonometric Function5/1 -> Product3/2
  Trigonometric Function/1 -> Product3/1
  Trigonometric Function6/1 -> Product3/3
  [i_theta] -> Trigonometric Function8/1, Trigonometric Function7/1
  [i_phi] -> Trigonometric Function9/1
  Trigonometric Function8/1 -> Product4/2
  Trigonometric Function7/1 -> Product4/1
  Trigonometric Function9/1 -> Product4/3
  [i_theta] -> Trigonometric Function11/1, Trigonometric Function10/1
  [i_phi] -> Trigonometric Function12/1
  Trigonometric Function11/1 -> Product5/2
  Trigonometric Function10/1 -> Product5/1
  Trigonometric Function12/1 -> Product5/3
  Product3/1 -> Gain5/1
  Product4/1 -> Gain6/1
  Product5/1 -> Gain7/1
  Gain4/1 -> Add3/1
  Gain5/1 -> Add3/2
  Gain6/1 -> Add3/3
  Gain7/1 -> Add3/4
  Add3/1 -> Product2/2

== system general_charger_2_precharge/Measurements/Power and angle calculations/AB-DQ Transform/Iab_dq/Iq Discretization Error Correction ==
  phi : Inport
  Q : Inport  Port=2
  wt : Inport  Port=3
  A : Inport  Port=4
  Add2 : Sum  Inputs=-+
  Add3 : Sum  Inputs=++-+
  Gain4 : Gain  Gain=0.000078956
  Gain5 : Gain  Gain=0.000078956
  Gain6 : Gain  Gain=0.012566039
  Gain7 : Gain  Gain=0.012566039
  Product{1,3..5} (4 alike) : Product  Inputs=3
  Product2 : Product
  Trigonometric Function{,1,3,5,7..9,11} (8 alike) : Trigonometry  Operator=cos
  Trigonometric Function{2,6,10,12} (4 alike) : Trigonometry
  Iq_corr : Outport
  wires:
  Add2/1 -> Iq_corr/1
  Product2/1 -> Add2/1
  Q/1 -> Add2/2
  A/1 -> Product2/1
  [i_theta] -> Trigonometric Function3/1, Trigonometric Function2/1
  [i_phi] -> Trigonometric Function1/1
  Trigonometric Function1/1 -> Product1/3
  Trigonometric Function2/1 -> Product1/1
  Trigonometric Function3/1 -> Product1/2
  Product1/1 -> Gain4/1
  [i_theta] -> Trigonometric Function5/1, Trigonometric Function/1
  [i_phi] -> Trigonometric Function6/1
  Trigonometric Function5/1 -> Product3/2
  Trigonometric Function/1 -> Product3/1
  Trigonometric Function6/1 -> Product3/3
  [i_theta] -> Trigonometric Function8/1, Trigonometric Function7/1
  [i_phi] -> Trigonometric Function9/1
  Trigonometric Function8/1 -> Product4/2
  Trigonometric Function7/1 -> Product4/1
  Trigonometric Function9/1 -> Product4/3
  [i_theta] -> Trigonometric Function11/1, Trigonometric Function10/1
  [i_phi] -> Trigonometric Function12/1
  Trigonometric Function11/1 -> Product5/2
  Trigonometric Function10/1 -> Product5/1
  Trigonometric Function12/1 -> Product5/3
  Product3/1 -> Gain5/1
  Product4/1 -> Gain6/1
  Product5/1 -> Gain7/1
  Gain4/1 -> Add3/1
  Gain5/1 -> Add3/2
  Gain6/1 -> Add3/3
  Gain7/1 -> Add3/4
  Add3/1 -> Product2/2
  wt/1 -> [i_theta]
  phi/1 -> [i_phi]

== system general_charger_2_precharge/Measurements/Power and angle calculations/AB-DQ Transform/Vab_dq/AB->DQ ==
  A : Inport
  wt : Inport  Port=2
  Add1 : Sum  Inputs=-+
  Add2 : Sum
  Delay : Delay  DelayLength=RSpC  SampleTime=abdq_Ts
  Product{1..4} (4 alike) : Product  RndMeth=Zero
  Trigonometric Function : Trigonometry
  Trigonometric Function1 : Trigonometry  Operator=cos
  Vd Discretization Error Correction : Subsystem
  Vq Discretization Error Correction : Subsystem
  D : Outport
  Q : Outport  Port=2
  wires:
  Trigonometric Function/1 -> Product1/1, Product2/1
  Product1/1 -> Add2/2
  Product4/1 -> Add2/1
  Product2/1 -> Add1/1
  A/1 -> Delay/1, Product4/1, Product2/2
  Trigonometric Function1/1 -> Product4/2, Product3/1
  Product3/1 -> Add1/2
  Delay/1 -> Product1/2, Product3/2  "B"
  wt/1 -> [theta], Trigonometric Function1/1, Trigonometric Function/1
  Add2/1 -> Vd Discretization Error Correction/3(D)  "Vd"
  Add1/1 -> Vq Discretization Error Correction/1(Q)
  [theta] -> Vq Discretization Error Correction/2(wt)
  [theta] -> Vd Discretization Error Correction/2(wt)
  Vd Discretization Error Correction/1(Vd_corr) -> D/1
  Vq Discretization Error Correction/1(Vq_corr) -> Q/1
  [Vpeak] -> Vq Discretization Error Correction/3(A)
  [Vpeak] -> Vd Discretization Error Correction/1(A)

== system general_charger_2_precharge/Measurements/Power and angle calculations/AB-DQ Transform/Vab_dq/PI1 ==
  in : Inport
  Add1 : Sum
  Add2 : Sum
  Ki : Gain  Gain=ki
  Kp : Gain  Gain=kp
  Tappe : simulink/Discrete/Tapped Delay  vinit=0.0  samptime=Ts_pi  NumDelays=1  DelayOrder=Oldest  includeCurrent=off
  Ts : Gain  Gain=Ts_pi
  integral saturation : Saturate  UpperLimit=int_sat_up  LowerLimit=int_sat_low  SampleTime=Ts_pi
  pi controller saturation : Saturate  UpperLimit=pi_sat_up  LowerLimit=pi_sat_low  SampleTime=Ts_pi
  out : Outport
  wires:
  Ts/1 -> Ki/1
  in/1 -> Kp/1, Ts/1  "vdc_error"
  Add1/1 -> integral saturation/1  "vdc_int_pi"
  Kp/1 -> Add2/2  "vdc_kp_pi"
  pi controller saturation/1 -> out/1
  Tappe/1 -> Add1/1
  Add2/1 -> pi controller saturation/1  "vdc_pi"
  Ki/1 -> Add1/2
  integral saturation/1 -> Add2/1, Tappe/1

== system general_charger_2_precharge/Measurements/Power and angle calculations/AB-DQ Transform/Vab_dq/PI4 ==
  in : Inport
  Add1 : Sum
  Add2 : Sum
  Ki : Gain  Gain=ki
  Kp : Gain  Gain=kp
  Tappe : simulink/Discrete/Tapped Delay  vinit=0.0  samptime=Ts_pi  NumDelays=1  DelayOrder=Oldest  includeCurrent=off
  Ts : Gain  Gain=Ts_pi
  integral saturation : Saturate  UpperLimit=int_sat_up  LowerLimit=int_sat_low  SampleTime=Ts_pi
  pi controller saturation : Saturate  UpperLimit=pi_sat_up  LowerLimit=pi_sat_low  SampleTime=Ts_pi
  out : Outport
  wires:
  Ts/1 -> Ki/1
  in/1 -> Kp/1, Ts/1  "vdc_error"
  Add1/1 -> integral saturation/1  "vdc_int_pi"
  Kp/1 -> Add2/2  "vdc_kp_pi"
  pi controller saturation/1 -> out/1
  Tappe/1 -> Add1/1
  Add2/1 -> pi controller saturation/1  "vdc_pi"
  Ki/1 -> Add1/2
  integral saturation/1 -> Add2/1, Tappe/1

== system general_charger_2_precharge/Measurements/Power and angle calculations/discrete low pass filter1/Ad(1,1)/q rounder16 ==
  in : Inport
  Gain9 : Gain  Gain=2^-q
  Idealized ADC quantizer : simulink_extras/Additional Discrete/Idealized ADC quantizer  NumberOfConverterBits=32  Vmin=-range  Vmax=range  OutputDataType=double  OutputNegativeValues=on
  out : Outport
  wires:
  in/1 -> Idealized ADC quantizer/1
  Idealized ADC quantizer/1 -> Gain9/1
  Gain9/1 -> out/1

== system general_charger_2_precharge/Measurements/Power and angle calculations/discrete low pass filter1/Ad(1,2)/q rounder16 ==
  in : Inport
  Gain9 : Gain  Gain=2^-q
  Idealized ADC quantizer : simulink_extras/Additional Discrete/Idealized ADC quantizer  NumberOfConverterBits=32  Vmin=-range  Vmax=range  OutputDataType=double  OutputNegativeValues=on
  out : Outport
  wires:
  in/1 -> Idealized ADC quantizer/1
  Idealized ADC quantizer/1 -> Gain9/1
  Gain9/1 -> out/1

== system general_charger_2_precharge/Measurements/Power and angle calculations/discrete low pass filter1/Ad(1,3)/q rounder16 ==
  in : Inport
  Gain9 : Gain  Gain=2^-q
  Idealized ADC quantizer : simulink_extras/Additional Discrete/Idealized ADC quantizer  NumberOfConverterBits=32  Vmin=-range  Vmax=range  OutputDataType=double  OutputNegativeValues=on
  out : Outport
  wires:
  in/1 -> Idealized ADC quantizer/1
  Idealized ADC quantizer/1 -> Gain9/1
  Gain9/1 -> out/1

== system general_charger_2_precharge/Measurements/Power and angle calculations/discrete low pass filter1/Ad(2,1)/q rounder16 ==
  in : Inport
  Gain9 : Gain  Gain=2^-q
  Idealized ADC quantizer : simulink_extras/Additional Discrete/Idealized ADC quantizer  NumberOfConverterBits=32  Vmin=-range  Vmax=range  OutputDataType=double  OutputNegativeValues=on
  out : Outport
  wires:
  in/1 -> Idealized ADC quantizer/1
  Idealized ADC quantizer/1 -> Gain9/1
  Gain9/1 -> out/1
